simulink model "RIEKF_test"  (R2017b)
settings: Solver=ode23  StartTime=0  StopTime=10  FixedStep=1e-5  EnableMultiTasking=on
InitFcn:
  | RIEKF_InitFcn;
values from neighbouring files (symbols this model uses):
  accel_true_bias_init = [0;0;0]    [RIEKF_InitFcn.m]
  accel_true_bias_noise_std = 0.0001*ones(3,1)    [RIEKF_InitFcn.m]
  accel_true_noise_std = 0.01*ones(3,1)    [RIEKF_InitFcn.m]
  EKF_SampleTime = 1/2000    (= 0.0005)    [RIEKF_InitFcn.m]
  EtherCat_SampleTime = 1/2000    (= 0.0005)    [RIEKF_InitFcn.m]
  gyro_true_bias_init = [0;0;0]    [RIEKF_InitFcn.m]
  gyro_true_bias_noise_std = 0.0001*ones(3,1)    [RIEKF_InitFcn.m]
  gyro_true_noise_std = 0.001*ones(3,1)    [RIEKF_InitFcn.m]
  landmark_measurement_frequency = 1/20    (= 0.05)    [RIEKF_InitFcn.m]
  landmark_positions = [0;0;0]    [RIEKF.m]    (also in RIEKF_InitFcn.m = [[1; 0;0;0],                       [2; 1;2;3],              )
  landmark_true_noise_std = 0.00*ones(3,1)    [RIEKF_InitFcn.m]
  VectorNav_SampleTime = 1/800    (= 0.00125)    [RIEKF_InitFcn.m]
undefined symbols (not defined in the file or in its folder): Case, Channel
libraries: simulink x6
settings Model: Creator=case  LastModifiedBy=DELL
settings SolverCC: ZeroCrossControl=DisableAll  InsertRTBMode=Always
settings DataIOCC: SaveOutput=off  SignalLogging=off  DSMLogging=off  SaveTime=off
settings OptimizationCC: DefaultParameterBehavior=Inlined  UseFloatMulNetSlope=on  InlineInvariantSignals=on  EfficientFloat2IntCast=on  LifeSpan=inf  SimCompilerOptimization=on  AccelVerboseBuild=on
settings DebuggingCC: ReadBeforeWriteMsg=DisableAll  WriteAfterWriteMsg=DisableAll  WriteAfterReadMsg=DisableAll  ParameterUnderflowMsg=error  ParameterTunabilityLossMsg=error  UniqueDataStoreMsg=error  AllowSymbolicDim=off  StrictBusMsg=ErrorOnBusTreatedAsVector  SFUnexpectedBacktrackingDiag=warning  SFNoUnconditionalDefaultTransitionDiag=warning  SFExecutionAtInitializationDiag=none
settings HardwareCC: TargetBitPerPointer=64  TargetBitPerSizeT=64  TargetBitPerPtrDiffT=64  TargetLongLongMode=on  TargetIntDivRoundTo=Zero  TargetEndianess=LittleEndian  TargetWordSize=64  TargetHWDeviceType=MATLAB Host  ProdEqTarget=off
settings ModelReferenceCC: UpdateModelReferenceTargets=IfOutOfDate  ModelReferenceNumInstancesAllowed=Zero  ModelReferenceMinAlgLoopOccurrences=on  PropagateSignalLabelsOutOfModel=off
settings RTWCC: Description=Generic Real-Time Target  RTWUseSimCustomCode=on  BuildConfiguration=Faster Runs  CheckMdlBeforeBuild=Warning
settings CodeAppCC: GenerateComments=off  SimulinkBlockComments=off
settings GRTTargetCC: MatFileLogging=off  MultiInstanceERTCode=on  CodeInterfacePackaging=Reusable function  SupportNonFinite=off  GenerateAllocFcn=on
settings ConfigComp: CovMetricSettings=dw  CovHtmlReporting=on  CovSaveCumulativeToWorkspaceVar=on  CovSaveSingleToWorkspaceVar=on  CovExternalEMLEnable=off
settings SimscapeCC: SimscapeNormalizeSystem=off
settings DiagnosticsConfigSet: SimMechanicsRigidlyBoundBlock=warning
settings ExplorerConfigSet: InternalSimMechanicsExplorerSettings="<ExplorerConfiguration><canonicalview>default</canonicalview><AnimationSetting><BasePlaybackSpeed>1.0</BasePlaybackSpeed><PlaybackSpeedFactor>1.0</PlaybackSpeedFactor></AnimationSetting><TilePanel><TileInfo><Tiles Columns=\"1\" Count=\"1\" Rows=\"1\"><Column Left=\"2\" Weight=\"1\"/><Column Left=\"1053\"/><Row Top=\"2\" Weight=\"1\"/><Row Top=\"486\"/><Tile Height=\"1\" Width=\"1\" X=\"0\" Y=\"0\"/></Tiles></TileInfo><SceneInfo><SceneViewer><BGColor><R>0.60000002384185791</R><G>0.60000002384185791</G><B>0.60000002384185791</B></BGColor><Camera><DoPerspective>on</DoPerspective><Position><X>1.5163613923952763</X><Y>-1.4988060678602755</Y><Z>0.66118837525886986</Z></Position><Center><X>0.016361392395276342</X><Y>0.0011939321397245184</Y><Z>0.16118837525886986</Z></Center><Up><X>0</X><Y>0</Y><Z>1</Z></Up><ViewLimDist>1</ViewLimDist><YLim>0.46630765815499858</YLim><XLim>1.0229317469421231</XLim></Camera></SceneViewer></SceneInfo></TilePanel><MechEditorPanel><Cameras><Camera><Id>Camera1</Id><Value><Name>Tracking Camera</Name><NativeCamera><PositionTrackingFeature>Cassie_V2_Simulation_Subsystem.Cassie_Multibody_Subsystem.Pelvis.Tracking_Camera.F</PositionTrackingFeature><CenterTrackingFeature>Cassie_V2_Simulation_Subsystem.Cassie_Multibody_Subsystem.Pelvis.Tracking_Camera_Target.F</CenterTrackingFeature><UpVectorTrackingFeature>Cassie_V2_Simulation_Subsystem.Cassie_Multibody_Subsystem.Pelvis.Tracking_Camera_Target.F</UpVectorTrackingFeature><CenterTrackingOrigin>on</CenterTrackingOrigin><UpVectorTrackingDirection>+Z</UpVectorTrackingDirection></NativeCamera></Value></Camera><Camera><Id>Camera2</Id><Value><Name>Fixed Camera</Name><NativeCamera><PositionTrackingFeature>Cassie_V2_Simulation_Subsystem.Cassie_Multibody_Subsystem.Pelvis.Fixed_Camera.F</PositionTrackingFeature><CenterTrackingFeature>Cassie_V2_Simulation_Subsystem.Cassie_Multibody_Subsystem.Pelvis.Fixed_Camera_Target.F</CenterTrackingFeature><UpVectorTrackingFeature>Cassie_V2_Simulation_Subsystem.Cassie_Multibody_Subsystem.Pelvis.Fixed_Camera_Target.F</UpVectorTrackingFeature><CenterTrackingOrigin>on</CenterTrackingOrigin><UpVectorTrackingDirection>+Z</UpVectorTrackingDirection></NativeCamera></Value></Camera></Cameras><GfxPanelCameraMap><MapElement CameraMLId=\"Camera1\" GfxPanelIndex=\"0\"/></GfxPanelCameraMap><VideoCreator><PlaybackSpeedRatio>1.0</PlaybackSpeedRatio><FrameRate>30</FrameRate><VideoFormat>Motion JPEG AVI</VideoFormat><FrameSize>auto</FrameSize></VideoCreator></MechEditorPanel></ExplorerConfiguration>"

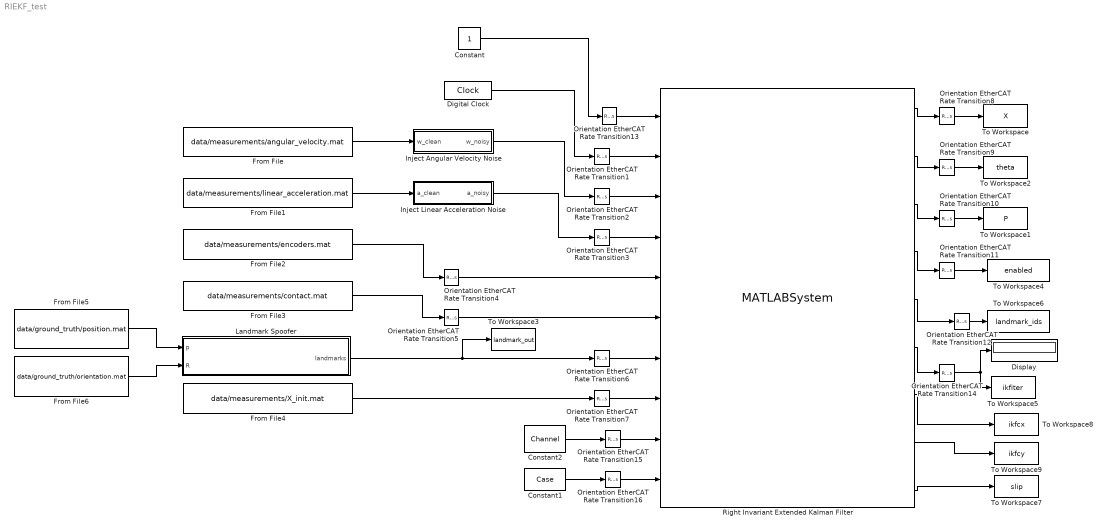
== system RIEKF_test ==
  Constant : Constant
  Constant1 : Constant  Value=Case
  Constant2 : Constant  Value=Channel
  Digital Clock : DigitalClock  SampleTime=EtherCat_SampleTime
  Display : Display
  From File : FromFile  FileName=data/measurements/angular_velocity.mat  SampleTime=0
  From File1 : FromFile  FileName=data/measurements/linear_acceleration.mat  SampleTime=0
  From File2 : FromFile  FileName=data/measurements/encoders.mat  SampleTime=0
  From File3 : FromFile  FileName=data/measurements/contact.mat  SampleTime=0
  From File4 : FromFile  FileName=data/measurements/X_init.mat  SampleTime=0
  From File5 : FromFile  FileName=data/ground_truth/position.mat  SampleTime=EKF_SampleTime
  From File6 : FromFile  FileName=data/ground_truth/orientation.mat  SampleTime=EKF_SampleTime
  Inject Angular Velocity Noise : Subsystem
  Inject Linear Acceleration Noise : Subsystem
  Landmark Spoofer : Subsystem
  Orientation EtherCAT Rate Transition{1..7,13,15..16} (10 alike) : RateTransition  Deterministic=off  OutPortSampleTime=EKF_SampleTime
  Orientation EtherCAT Rate Transition{8..12,14} (6 alike) : RateTransition  Deterministic=off  OutPortSampleTime=EtherCat_SampleTime
  Right Invariant Extended Kalman Filter : MATLABSystem  System=RIEKF  static_bias_initialization=static_bias_initialization  ekf_update_enabled=ekf_update_enabled  enable_kinematic_measurements=enable_kinematic_measurements  enable_landmark_measurements=enable_landmark_measurements  enable_static_landmarks=enable_static_landmarks  gyro_noise_std=gyro_noise_std  gyro_bias_noise_std=gyro_bias_noise_std  accel_noise_std=accel_noise_std  accel_bias_noise_std=accel_bias_noise_std  contact_noise_std=contact_noise_std  encoder_noise_std=encoder_noise_std  landmark_noise_std=landmark_noise_std  gyro_bias_init=gyro_bias_init  accel_bias_init=accel_bias_init  prior_base_pose_std=prior_base_pose_std  prior_base_velocity_std=prior_base_velocity_std  prior_contact_position_std=prior_contact_position_std  prior_gyro_bias_std=prior_gyro_bias_std  prior_accel_bias_std=prior_accel_bias_std  prior_forward_kinematics_std=prior_forward_kinematics_std  landmark_positions=landmark_positions  SimulateUsing=Interpreted execution
      mask Type: RIEKF
      mask Display:
      | disp('RIEKF');
      | port_label('input',1,'enable');
      | port_label('input',2,'t');
      | port_label('input',3,'w');
      | port_label('input',4,'a');
      | port_label('input',5,'encoders');
      | port_label('input',6,'contact');
      | port_label('input',7,'landmarks');
      | port_label('input',8,'X_init');
      | port_label('input',9,'Channel');
      | port_label('input',10,'Case');
      | port_label('output',1,'X');
      | port_label('output',2,'theta');
      | port_label('output',3,'P');
      | port_label('output',4,'enabled');
      | port_label('output',5,'landmark_ids');
      | port_label('output',6,'ikfiter');
      | port_label('output',7,'ikfcx');
      | port_label('output',8,'ikfcy');
      | port_label('output',9,'slipn');
  To Workspace : ToWorkspace  VariableName=X  SaveFormat=Structure With Time  SampleTime=-1
  To Workspace1 : ToWorkspace  VariableName=P  SaveFormat=Structure With Time  SampleTime=-1
  To Workspace2 : ToWorkspace  VariableName=theta  SaveFormat=Structure With Time  SampleTime=-1
  To Workspace3 : ToWorkspace  VariableName=landmark_out  SaveFormat=Structure With Time  SampleTime=-1
  To Workspace4 : ToWorkspace  VariableName=enabled  SaveFormat=Structure With Time  SampleTime=-1
  To Workspace5 : ToWorkspace  VariableName=ikfiter  SaveFormat=Structure With Time  SampleTime=-1
  To Workspace6 : ToWorkspace  VariableName=landmark_ids  SaveFormat=Structure With Time  SampleTime=-1
  To Workspace7 : ToWorkspace  VariableName=slip  SaveFormat=Structure With Time  SampleTime=-1
  To Workspace8 : ToWorkspace  VariableName=ikfcx  SaveFormat=Structure With Time  SampleTime=-1
  To Workspace9 : ToWorkspace  VariableName=ikfcy  SaveFormat=Structure With Time  SampleTime=-1
  wires:
  From File/1 -> Inject Angular Velocity Noise/1(w_clean)
  Constant/1 -> Orientation EtherCAT Rate Transition13/1
  Digital Clock/1 -> Orientation EtherCAT Rate Transition1/1
  From File1/1 -> Inject Linear Acceleration Noise/1(a_clean)
  From File2/1 -> Orientation EtherCAT Rate Transition4/1
  From File4/1 -> Orientation EtherCAT Rate Transition7/1
  Landmark Spoofer/1(landmarks) -> Orientation EtherCAT Rate Transition6/1, To Workspace3/1
  Right Invariant Extended Kalman Filter/4 -> Orientation EtherCAT Rate Transition11/1
  Right Invariant Extended Kalman Filter/5 -> Orientation EtherCAT Rate Transition12/1
  Right Invariant Extended Kalman Filter/3 -> Orientation EtherCAT Rate Transition10/1
  Right Invariant Extended Kalman Filter/2 -> Orientation EtherCAT Rate Transition9/1
  Right Invariant Extended Kalman Filter/1 -> Orientation EtherCAT Rate Transition8/1
  Orientation EtherCAT Rate Transition13/1 -> Right Invariant Extended Kalman Filter/1
  Orientation EtherCAT Rate Transition1/1 -> Right Invariant Extended Kalman Filter/2
  Orientation EtherCAT Rate Transition2/1 -> Right Invariant Extended Kalman Filter/3
  Orientation EtherCAT Rate Transition3/1 -> Right Invariant Extended Kalman Filter/4
  Orientation EtherCAT Rate Transition5/1 -> Right Invariant Extended Kalman Filter/6
  Orientation EtherCAT Rate Transition6/1 -> Right Invariant Extended Kalman Filter/7
  Orientation EtherCAT Rate Transition7/1 -> Right Invariant Extended Kalman Filter/8
  Inject Angular Velocity Noise/1(w_noisy) -> Orientation EtherCAT Rate Transition2/1
  Inject Linear Acceleration Noise/1(a_noisy) -> Orientation EtherCAT Rate Transition3/1
  Orientation EtherCAT Rate Transition8/1 -> To Workspace/1
  Orientation EtherCAT Rate Transition9/1 -> To Workspace2/1
  From File5/1 -> Landmark Spoofer/1(p)
  From File6/1 -> Landmark Spoofer/2(R)
  Orientation EtherCAT Rate Transition12/1 -> To Workspace6/1
  Orientation EtherCAT Rate Transition10/1 -> To Workspace1/1
  Orientation EtherCAT Rate Transition11/1 -> To Workspace4/1
  From File3/1 -> Orientation EtherCAT Rate Transition5/1
  Orientation EtherCAT Rate Transition4/1 -> Right Invariant Extended Kalman Filter/5
  Right Invariant Extended Kalman Filter/6 -> Orientation EtherCAT Rate Transition14/1
  Orientation EtherCAT Rate Transition14/1 -> To Workspace5/1, Display/1
  Right Invariant Extended Kalman Filter/8 -> To Workspace9/1
  Right Invariant Extended Kalman Filter/7 -> To Workspace8/1
  Right Invariant Extended Kalman Filter/9 -> To Workspace7/1
  Orientation EtherCAT Rate Transition15/1 -> Right Invariant Extended Kalman Filter/9
  Orientation EtherCAT Rate Transition16/1 -> Right Invariant Extended Kalman Filter/10
  Constant1/1 -> Orientation EtherCAT Rate Transition16/1
  Constant2/1 -> Orientation EtherCAT Rate Transition15/1

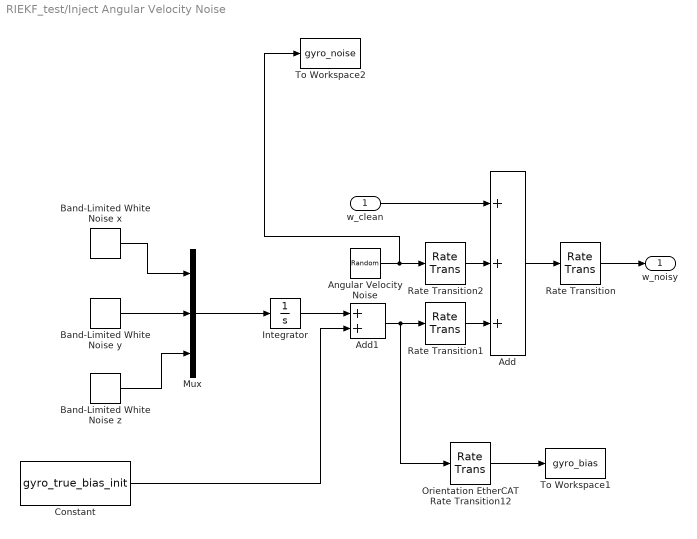
== system RIEKF_test/Inject Angular Velocity Noise ==
  w_clean : Inport
  Add : Sum  Inputs=+++
  Add1 : Sum
  Angular Velocity Noise : RandomNumber  Mean=[0;0;0]  Variance=[gyro_true_noise_std(1)^2; gyro_true_noise_std(2)^2; gyro_true_noise_std(3)^2]  Seed=[7;8;9]  SampleTime=VectorNav_SampleTime
  Band-Limited White Noise x : simulink/Sources/Band-Limited White Noise  Cov=[gyro_true_bias_noise_std(1)^2]  Ts=EtherCat_SampleTime  seed=[1]
  Band-Limited White Noise y : simulink/Sources/Band-Limited White Noise  Cov=[gyro_true_bias_noise_std(2)^2]  Ts=EtherCat_SampleTime  seed=[2]
  Band-Limited White Noise z : simulink/Sources/Band-Limited White Noise  Cov=[gyro_true_bias_noise_std(3)^2]  Ts=EtherCat_SampleTime  seed=[3]
  Constant : Constant  Value=gyro_true_bias_init
  Integrator : Integrator  InitialCondition=[0;0;0]
  Mux : Mux  Inputs=3
  Orientation EtherCAT Rate Transition12 : RateTransition  Deterministic=off  OutPortSampleTime=EtherCat_SampleTime
  Rate Transition : RateTransition  OutPortSampleTime=EtherCat_SampleTime
  Rate Transition1 : RateTransition  Deterministic=off  OutPortSampleTime=EtherCat_SampleTime
  Rate Transition2 : RateTransition  Deterministic=off  OutPortSampleTime=EtherCat_SampleTime
  To Workspace1 : ToWorkspace  VariableName=gyro_bias  SaveFormat=Timeseries  SampleTime=-1
  To Workspace2 : ToWorkspace  VariableName=gyro_noise  SaveFormat=Structure With Time  SampleTime=-1
  w_noisy : Outport
  wires:
  Orientation EtherCAT Rate Transition12/1 -> To Workspace1/1
  Rate Transition2/1 -> Add/2
  Rate Transition1/1 -> Add/3
  Constant/1 -> Add1/2
  Add1/1 -> Rate Transition1/1, Orientation EtherCAT Rate Transition12/1
  Angular Velocity Noise/1 -> Rate Transition2/1, To Workspace2/1
  Integrator/1 -> Add1/1
  Band-Limited White Noise x/1 -> Mux/1
  Band-Limited White Noise y/1 -> Mux/2
  Band-Limited White Noise z/1 -> Mux/3
  Mux/1 -> Integrator/1
  Rate Transition/1 -> w_noisy/1
  Add/1 -> Rate Transition/1
  w_clean/1 -> Add/1

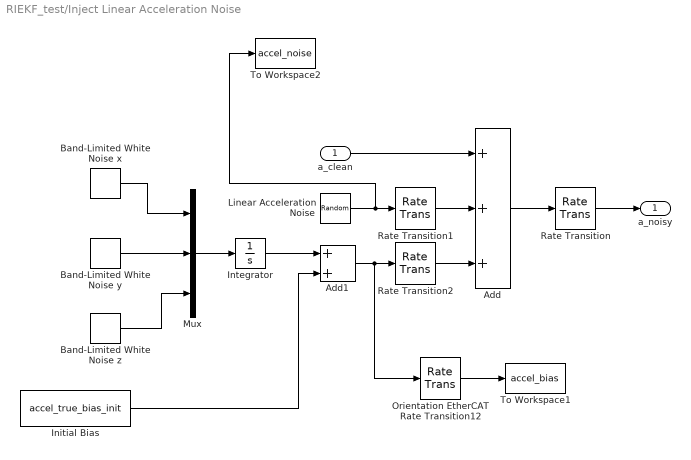
== system RIEKF_test/Inject Linear Acceleration Noise ==
  a_clean : Inport
  Add : Sum  Inputs=+++
  Add1 : Sum
  Band-Limited White Noise x : simulink/Sources/Band-Limited White Noise  Cov=[accel_true_bias_noise_std(1)^2]  Ts=EtherCat_SampleTime  seed=[4]
  Band-Limited White Noise y : simulink/Sources/Band-Limited White Noise  Cov=[accel_true_bias_noise_std(2)^2]  Ts=EtherCat_SampleTime  seed=[5]
  Band-Limited White Noise z : simulink/Sources/Band-Limited White Noise  Cov=[accel_true_bias_noise_std(3)^2]  Ts=EtherCat_SampleTime  seed=[6]
  Initial Bias : Constant  Value=accel_true_bias_init
  Integrator : Integrator  InitialCondition=[0;0;0]
  Linear Acceleration Noise : RandomNumber  Mean=[0;0;0]  Variance=[accel_true_noise_std(1)^2; accel_true_noise_std(2)^2; accel_true_noise_std(3)^2]  Seed=[10;11;12]  SampleTime=VectorNav_SampleTime
  Mux : Mux  Inputs=3
  Orientation EtherCAT Rate Transition12 : RateTransition  Deterministic=off  OutPortSampleTime=EtherCat_SampleTime
  Rate Transition : RateTransition  OutPortSampleTime=EtherCat_SampleTime
  Rate Transition1 : RateTransition  Deterministic=off  OutPortSampleTime=EtherCat_SampleTime
  Rate Transition2 : RateTransition  Deterministic=off  OutPortSampleTime=EtherCat_SampleTime
  To Workspace1 : ToWorkspace  VariableName=accel_bias  SaveFormat=Timeseries  SampleTime=-1
  To Workspace2 : ToWorkspace  VariableName=accel_noise  SaveFormat=Structure With Time  SampleTime=-1
  a_noisy : Outport
  wires:
  Rate Transition/1 -> a_noisy/1
  Orientation EtherCAT Rate Transition12/1 -> To Workspace1/1
  Rate Transition2/1 -> Add/3
  Rate Transition1/1 -> Add/2
  Add1/1 -> Rate Transition2/1, Orientation EtherCAT Rate Transition12/1
  Initial Bias/1 -> Add1/2
  a_clean/1 -> Add/1
  Linear Acceleration Noise/1 -> Rate Transition1/1, To Workspace2/1
  Band-Limited White Noise x/1 -> Mux/1
  Band-Limited White Noise y/1 -> Mux/2
  Band-Limited White Noise z/1 -> Mux/3
  Mux/1 -> Integrator/1
  Integrator/1 -> Add1/1
  Add/1 -> Rate Transition/1

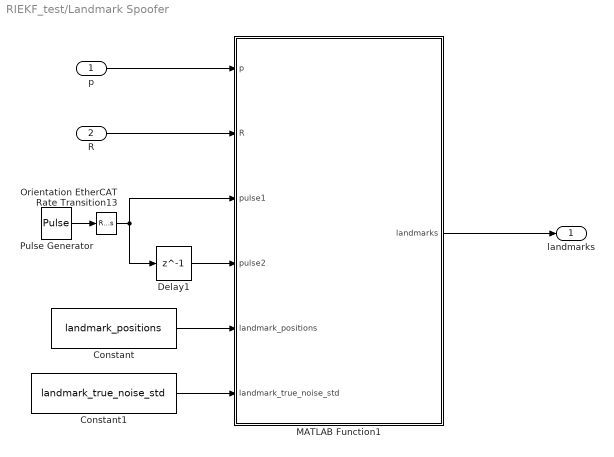
== system RIEKF_test/Landmark Spoofer ==
  p : Inport
  R : Inport  Port=2
  Constant : Constant  Value=landmark_positions
  Constant1 : Constant  Value=landmark_true_noise_std
  Delay1 : Delay  DelayLength=1  InitialCondition=0
  MATLAB Function1 : MATLAB Function  TreatAsAtomicUnit=on
  Orientation EtherCAT Rate Transition13 : RateTransition  Deterministic=off  OutPortSampleTime=EKF_SampleTime
  Pulse Generator : DiscretePulseGenerator  PulseType=Time based  Period=landmark_measurement_frequency  PulseWidth=5
  landmarks : Outport
  wires:
  Pulse Generator/1 -> Orientation EtherCAT Rate Transition13/1
  MATLAB Function1/1(landmarks) -> landmarks/1
  Delay1/1 -> MATLAB Function1/4(pulse2)
  Orientation EtherCAT Rate Transition13/1 -> Delay1/1, MATLAB Function1/3(pulse1)
  Constant/1 -> MATLAB Function1/5(landmark_positions)
  Constant1/1 -> MATLAB Function1/6(landmark_true_noise_std)
  p/1 -> MATLAB Function1/1(p)
  R/1 -> MATLAB Function1/2(R)

== matlab function RIEKF_test/Landmark Spoofer/MATLAB Function1 ==
  data: p input; R input; landmarks output size=[4,10]; pulse1 input; pulse2 input; landmark_positions input; landmark_true_noise_std input
function landmarks = SpoofLandmarks(p, R, pulse1, pulse2, landmark_positions, landmark_true_noise_std)

% Trigger of rising edge of pulse
if pulse1 && ~pulse2
    enable = true;
else
    enable = false;
end

% Initialize landmarks
landmarks = [];

% Compute landmark measurements
if enable
    % Compute World to IMU rotation matrix
    %R = Angles.Quaternion_to_Rotation(orientation([2;3;4;1]))';
    
    % Compute landmark measurments
    % {I}_p_{IL} = R_{WB}^T * ({W}_p_{WL} - {W}_p_{WI})
    N = size(landmark_positions,2);
    indices = randsample(N,randi(N));
    while(~isempty(indices))
        measurement = R'*(landmark_positions(2:4,indices(end)) - p) + landmark_true_noise_std.*randn(3,1); % 7 landmark with known position
        landmarks = horzcat(landmarks, [landmark_positions(1,indices(end)); measurement]);
        indices(end) = [];
    end
end

end
